simulink model "hdv_hydroelectropowertrain_model"  (R2023b)
settings: Solver=ode1be  StartTime=0.0  StopTime=simulation_length  FixedStep=tsample  MaxStep=tsample
values from neighbouring files (symbols this model uses):
  alpha = 35    [init_model.m]
  Apump = [0 1; 0 0]    [init_model.m]
  available_torque = torque_base+torque_friction_base    [init_model.m]
  Bpump = [0 1]'    [init_model.m]
  btheta_shaft = 2e2    (= 200)    [init_model.m]
  C1 = 10    [init_model.m]
  consumption = [consumption_1, consumption_2, consumption_3, consumption_4,          consumption_5, consumption_6, consumption_7, consumption_8,          consumption_9, consumption_10, consumption_11, consumption_12,          consumption_13, consumption_14, consumption_15, consumption_16          ]    [ic_engine_data.m]
  Cpump = [k 0]    [init_model.m]
  dp_lim = 400    [init_model.m]
  E0 = 3.685    [init_model.m]
  E1 = 0.2156    [init_model.m]
  E2 = 0    [init_model.m]
  E3 = 0    [init_model.m]
  E_1 = -1.031    [init_model.m]
  Elog = -0.05    [init_model.m]
  eta_v_m = 0.98    [init_model.m]
  eta_v_p = 0.97    [init_model.m]
  ki_dp_comp = 1/dp_lim    (= 0.0025)    [init_model.m]
  ki_te_comp = 2/te_lim    [init_model.m]
  kp_ctrl_m = 1    [init_model.m]
  kp_dp_comp = 0.5/dp_lim    (= 0.00125)    [init_model.m]
  kp_te_comp = 1/te_lim    [init_model.m]
  Kpump = acker(Apump,Bpump,poles)    [init_model.m]
  load_blade_enable = 0    [init_model.m]
  Lpump = acker(Apump',Cpump',pole_so)'    [init_model.m]
  M = 125    [init_model.m]
  Ncell = 185    [init_model.m]
  Npump = -1/(Cpump*inv(Apump-Bpump*Kpump)*Bpump)    [init_model.m]
  omega_e_rpm_ref = 1700    [init_model.m]
  omega_l_max_rpm = omega_l_max/(2*pi)*60    (= 50.3075969543)    [init_model.m]
  q1Kalman = tsample^2*1e-2    (= 1e-08)    [init_model.m]
  q2Kalman = tsample^1*1e-1    (= 0.0001)    [init_model.m]
  q3Kalman = 0    [init_model.m]
  Qhr = 400    [init_model.m]
  R0 = 0.015    [init_model.m]
  R1 = 0.015    [init_model.m]
  R_tg = 1.16/2    (= 0.58)    [init_model.m]
  rKalman = 1    [init_model.m]
  rpm_base = [620 700 800 900 1000 1100 1200 1300 1400 1500 1600 1700 1800      1900 2000 2100]    [ic_engine_data.m]
  rpm_consumption = rpm_base    [ic_engine_data.m]
  simulation_length = 245    [init_model.m]
  tau_load = 75e3    (= 75000)    [init_model.m]
  tau_load_max = 1600*41.4    (= 66240)    [init_model.m]
  Tc = tsample    (= 0.001)    [init_model.m]
  torque_base = [max(torque_16_data) max(torque_15_data) max(torque_14_data)      max(torque_13_data) max(torque_12_data) max(torque_11_data)      max(torque_10_data) max(torque_9_data) max(torque_8_data)      max(torque_7_data) max(torque_6_data) max(torque_5_data)      max(torque_4_data) max(torque_3_data) max(torque_2_data)      max(torque_1_data)]    [ic_engine_data.m]
  torque_consumption = torque_reference    [ic_engine_data.m]
  torque_friction_base = -(rpm_base./60*2*pi)*0.25-(rpm_base./60*2*pi).^2*5.2e-4    [ic_engine_data.m]
  tsample = 1e-3    (= 0.001)    [init_model.m]
  v_track1_ref = 8    [init_model.m]
  v_track2_ref = 8    [init_model.m]
  valve_mmorifice_max = 2.75    [init_model.m]
  xv_m_max = 1.2    [init_model.m]
undefined symbols (not defined in the file or in its folder): magnitude
libraries: fl_lib x381, nesl_utility x162, linear_swashplate_ctrl_lib x8, flexshaft_lib x5, bichamber_piston_lib x5, variable_displacement_motor_lib x4, variable_displacement_pump_lib x4, fixed_displacement_pump_lib x4, relief_valve_lib x4, inverse_shuttle_valve_lib x4, hydrostatic_threeway_valve_bichamber_piston_lib x4, hydrostatic_fourway_valve_bichamber_piston_lib x4
(part 2 of 9)

== system hdv_hydroelectropowertrain_model/Vehicle Control System/direction_lineLT ==
  In1 : Inport
  Abs1 : Abs  SaturateOnIntegerOverflow=off
  Product : Product
  Out1 : Outport
  wires:
  [direction_LT] -> Product/2
  In1/1 -> Abs1/1
  Product/1 -> Out1/1
  Abs1/1 -> Product/1

== system hdv_hydroelectropowertrain_model/Vehicle Control System/direction_lineRT ==
  In1 : Inport
  Abs : Abs  SaturateOnIntegerOverflow=off
  Product : Product
  Out1 : Outport
  wires:
  Product/1 -> Out1/1
  In1/1 -> Abs/1
  [direction_RT] -> Product/2
  Abs/1 -> Product/1

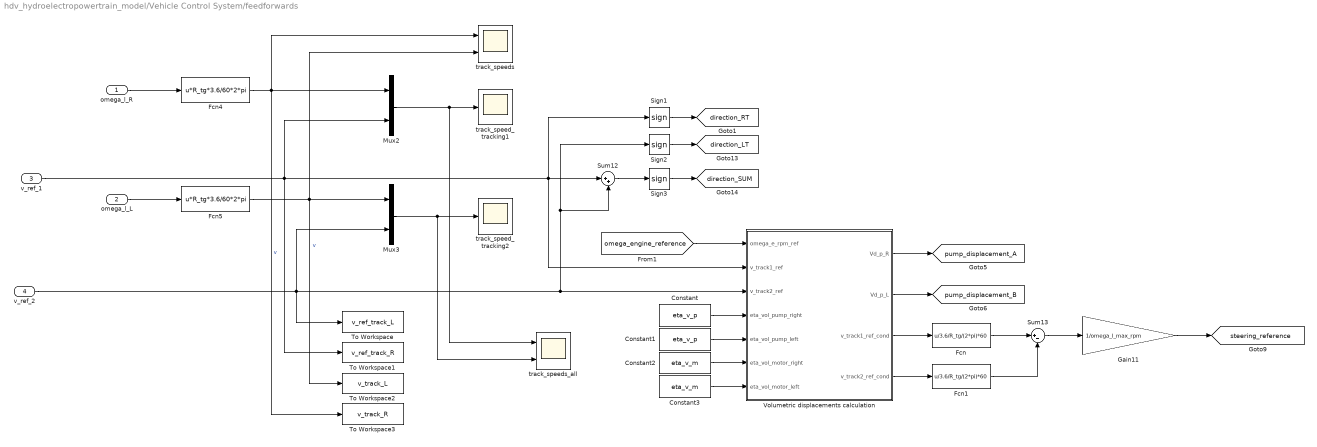
== system hdv_hydroelectropowertrain_model/Vehicle Control System/feedforwards ==
  omega_l_R : Inport
  omega_l_L : Inport  Port=2
  v_ref_1 : Inport  Port=3
  v_ref_2 : Inport  Port=4
  Constant : Constant  Value=eta_v_p
  Constant1 : Constant  Value=eta_v_p
  Constant2 : Constant  Value=eta_v_m
  Constant3 : Constant  Value=eta_v_m
  Fcn : Fcn  Expr=u/3.6/R_tg/(2*pi)*60
  Fcn1 : Fcn  Expr=u/3.6/R_tg/(2*pi)*60
  Fcn4 : Fcn  Expr=u*R_tg*3.6/60*2*pi
  Fcn5 : Fcn  Expr=u*R_tg*3.6/60*2*pi
  Gain11 : Gain  Gain=1/omega_l_max_rpm
  Mux2 : Mux  Inputs=2
  Mux3 : Mux  Inputs=2
  Sign1 : Signum
  Sign2 : Signum
  Sign3 : Signum
  Sum12 : Sum  Inputs=|++
  Sum13 : Sum  Inputs=|+-
  To Workspace : ToWorkspace  VariableName=v_ref_track_L  SampleTime=Tc
      settings: MaxDataPoints=Nc
  To Workspace1 : ToWorkspace  VariableName=v_ref_track_R  SampleTime=Tc
      settings: MaxDataPoints=Nc
  To Workspace2 : ToWorkspace  VariableName=v_track_L  SampleTime=Tc
      settings: MaxDataPoints=Nc
  To Workspace3 : ToWorkspace  VariableName=v_track_R  SampleTime=Tc
      settings: MaxDataPoints=Nc
  Volumetric displacements calculation : MATLAB Function  TreatAsAtomicUnit=on
  track_speed_tracking1 : Scope
  track_speed_tracking2 : Scope
  track_speeds : Scope  NumInputPorts=2
  track_speeds_all : Scope  NumInputPorts=2
  tag scope: direction_LT=global, direction_RT=global, direction_SUM=global, pump_displacement_A=global, pump_displacement_B=global, steering_reference=global
  wires:
  Constant3/1 -> Volumetric displacements calculation/7(eta_vol_motor_left)
  [omega_engine_reference] -> Volumetric displacements calculation/1(omega_e_rpm_ref)
  v_ref_2/1 -> To Workspace/1, Sign2/1, Sum12/2, Volumetric displacements calculation/3(v_track2_ref), Mux3/2
  v_ref_1/1 -> Mux2/2, To Workspace1/1, Volumetric displacements calculation/2(v_track1_ref), Sum12/1, Sign1/1
  Fcn/1 -> Sum13/1
  Constant/1 -> Volumetric displacements calculation/4(eta_vol_pump_right)
  Volumetric displacements calculation/4(v_track2_ref_cond) -> Fcn1/1
  Fcn5/1 -> To Workspace2/1, Mux3/1, track_speeds/2  "v"
  Constant1/1 -> Volumetric displacements calculation/5(eta_vol_pump_left)
  Sum13/1 -> Gain11/1
  Volumetric displacements calculation/3(v_track1_ref_cond) -> Fcn/1
  Sign1/1 -> [direction_RT]
  Fcn4/1 -> Mux2/1, track_speeds/1, To Workspace3/1  "v"
  Volumetric displacements calculation/1(Vd_p_R) -> [pump_displacement_A]
  Volumetric displacements calculation/2(Vd_p_L) -> [pump_displacement_B]
  omega_l_R/1 -> Fcn4/1
  Gain11/1 -> [steering_reference]
  Sign2/1 -> [direction_LT]
  Sum12/1 -> Sign3/1
  Sign3/1 -> [direction_SUM]
  Constant2/1 -> Volumetric displacements calculation/6(eta_vol_motor_right)
  Mux3/1 -> track_speeds_all/2, track_speed_tracking2/1
  Fcn1/1 -> Sum13/2
  Mux2/1 -> track_speeds_all/1, track_speed_tracking1/1
  omega_l_L/1 -> Fcn5/1

== system hdv_hydroelectropowertrain_model/Vehicle Control System/lineA_compensations ==
  Abs : Abs  SaturateOnIntegerOverflow=off
  Gain7 : Gain  Gain=-1
  Saturation Dynamic : simulink/Discontinuities/Saturation Dynamic  OutMin=[]  OutMax=[]  OutDataTypeStr=Inherit: Same as second input  OutDataType=fixdt(1, 16)  OutScaling=2^-10  DoSatur=off
  Sum13 : Sum  Inputs=++|
  compRT : Scope  NumInputPorts=2
  direction_RT : Subsystem
  displacement_compensation : Outport
  wires:
  Saturation Dynamic/1 -> displacement_compensation/1
  Sum13/1 -> Saturation Dynamic/2
  Gain7/1 -> compRT/2, Saturation Dynamic/3
  [compensation_pressureA] -> Sum13/1
  [compensation_engine] -> direction_RT/1(In1)
  direction_RT/1(ETComp) -> Sum13/2  "engine torque compensation"
  [pump_displacement_A] -> Abs/1
  Abs/1 -> Saturation Dynamic/1, compRT/1, Gain7/1

== system hdv_hydroelectropowertrain_model/Vehicle Control System/lineB_compensations  ==
  Abs : Abs  SaturateOnIntegerOverflow=off
  Gain7 : Gain  Gain=-1
  Saturation Dynamic : simulink/Discontinuities/Saturation Dynamic  OutMin=[]  OutMax=[]  OutDataTypeStr=Inherit: Same as second input  OutDataType=fixdt(1, 16)  OutScaling=2^-10  DoSatur=off
  Sum12 : Sum  Inputs=|++
  compLT : Scope  NumInputPorts=2
  direction_LT : Subsystem
  displacement_compensation : Outport
  wires:
  [compensation_pressureB] -> Sum12/2
  Gain7/1 -> compLT/2, Saturation Dynamic/3
  [compensation_engine] -> direction_LT/1(In1)
  direction_LT/1(ETComp) -> Sum12/1  "engine torque compensation"
  [pump_displacement_B] -> Abs/1
  Sum12/1 -> Saturation Dynamic/2
  Saturation Dynamic/1 -> displacement_compensation/1
  Abs/1 -> Saturation Dynamic/1, compLT/1, Gain7/1

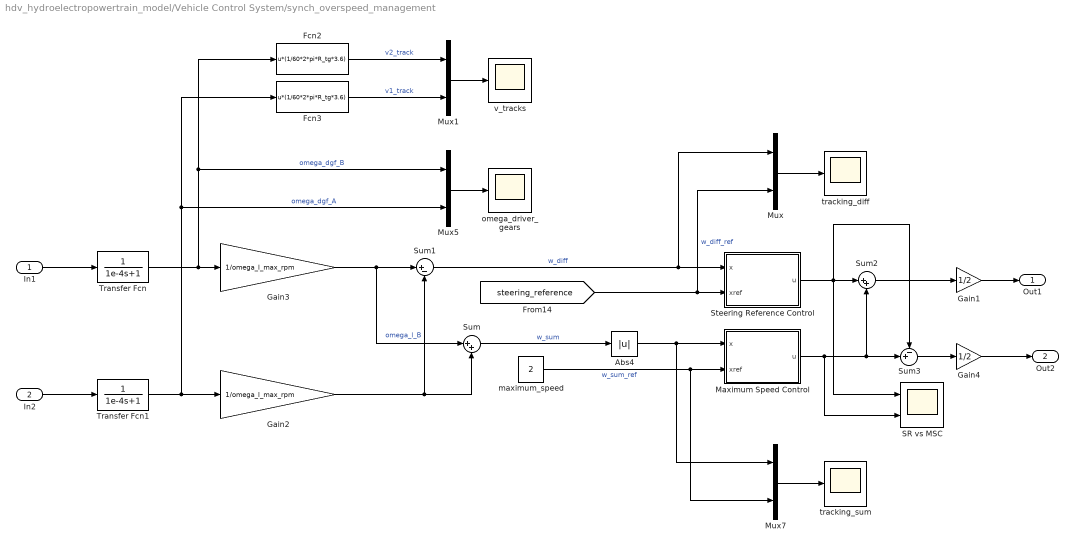
== system hdv_hydroelectropowertrain_model/Vehicle Control System/synch_overspeed_management ==
  In1 : Inport
  In2 : Inport  Port=2
  Abs4 : Abs  SaturateOnIntegerOverflow=off
  Fcn2 : Fcn  Expr=u*(1/60*2*pi*R_tg*3.6)
  Fcn3 : Fcn  Expr=u*(1/60*2*pi*R_tg*3.6)
  Gain1 : Gain  Gain=1/2
  Gain2 : Gain  Gain=1/omega_l_max_rpm
  Gain3 : Gain  Gain=1/omega_l_max_rpm
  Gain4 : Gain  Gain=1/2
  Maximum Speed Control : Subsystem  mask{kp=0.25/2, ki=4/2, ts=tsample, sat_pos=0, sat_neg=-3.28}
  Mux{,1,5,7} (4 alike) : Mux  Inputs=2
  SR vs MSC : Scope  NumInputPorts=2
  Steering Reference Control : Subsystem  mask{kp=0.125 %0.5, ki=2 %8, ts=tsample, sat_pos=3.28, sat_neg=-3.28}
  Sum : Sum  Inputs=|++
  Sum1 : Sum  Inputs=|+-
  Sum2 : Sum  Inputs=|++
  Sum3 : Sum  Inputs=-+|
  Transfer Fcn : TransferFcn  Denominator=[1e-4 1]
  Transfer Fcn1 : TransferFcn  Denominator=[1e-4 1]
  maximum_speed : Constant  Value=2
  omega_driver_gears : Scope
  tracking_diff : Scope
  tracking_sum : Scope
  v_tracks : Scope
  Out1 : Outport
  Out2 : Outport  Port=2
  wires:
  Mux7/1 -> tracking_sum/1
  Sum/1 -> Abs4/1  "w_sum"
  Gain3/1 -> Sum/1, Sum1/1
  Mux1/1 -> v_tracks/1
  maximum_speed/1 -> Maximum Speed Control/2(xref), Mux7/2  "w_sum_ref"
  Sum3/1 -> Gain4/1
  Sum1/1 -> Mux/1, Steering Reference Control/1(x)  "w_diff"
  Transfer Fcn/1 -> Fcn2/1, Mux5/1, Gain3/1  "omega_dgf_B"
  Maximum Speed Control/1(u) -> SR vs MSC/2, Sum2/2, Sum3/2
  Gain2/1 -> Sum1/2, Sum/2  "omega_l_B"
  In1/1 -> Transfer Fcn/1
  Mux/1 -> tracking_diff/1
  Gain1/1 -> Out1/1
  Sum2/1 -> Gain1/1
  Mux5/1 -> omega_driver_gears/1
  Abs4/1 -> Mux7/1, Maximum Speed Control/1(x)
  Fcn3/1 -> Mux1/2  "v1_track"
  [steering_reference] -> Mux/2, Steering Reference Control/2(xref)  "w_diff_ref"
  Steering Reference Control/1(u) -> Sum3/1, SR vs MSC/1, Sum2/1
  Transfer Fcn1/1 -> Fcn3/1, Mux5/2, Gain2/1  "omega_dgf_A"
  Fcn2/1 -> Mux1/1  "v2_track"
  Gain4/1 -> Out2/1
  In2/1 -> Transfer Fcn1/1

== system hdv_hydroelectropowertrain_model/Vehicle Control System/tracks references ==
  Manual Switch : ManualSwitch
  Manual Switch1 : ManualSwitch  CurrentSetting=0
  Repeating Sequence Stair1 : simulink/Sources/Repeating Sequence Stair  OutValues=[v_track2_ref -v_track2_ref v_track2_ref -v_track2_ref v_track2_ref -v_track2_ref].'  tsamp=floor(simulation_length/6)  OutMin=[]  OutMax=[]  OutDataTypeStr=double  OutputDataTypeScalingMode=double  OutDataType=fixdt(0,8)  ConRadixGroup=Best Precision: Vector-wise  OutScaling=2^-12
  Repeating Sequence Stair2 : simulink/Sources/Repeating Sequence Stair  OutValues=[v_track1_ref -v_track1_ref v_track1_ref -v_track1_ref v_track1_ref -v_track1_ref].'  tsamp=floor(simulation_length/6)  OutMin=[]  OutMax=[]  OutDataTypeStr=double  OutputDataTypeScalingMode=double  OutDataType=fixdt(0,8)  ConRadixGroup=Best Precision: Vector-wise  OutScaling=2^-12
  Sum : Sum  Inputs=|++
  Sum1 : Sum  Inputs=++|
  v_track1_ref : Step  Time=10  After=v_track1_ref  SampleTime=0
  v_track1_ref1 : Step  Time=simulation_length/2  After=-2*v_track1_ref  SampleTime=0
  v_track2_ref : Step  Time=10  After=v_track2_ref  SampleTime=0
  v_track2_ref1 : Step  Time=simulation_length/2  After=-2*v_track2_ref  SampleTime=0
  speed_track_1_ref : Outport
  speed_track_2_ref : Outport  Port=2
  wires:
  v_track1_ref1/1 -> Sum1/1
  v_track2_ref1/1 -> Sum/2
  v_track1_ref/1 -> Sum1/2
  v_track2_ref/1 -> Sum/1
  Manual Switch/1 -> speed_track_1_ref/1
  Manual Switch1/1 -> speed_track_2_ref/1
  Sum1/1 -> Manual Switch/2
  Sum/1 -> Manual Switch1/1
  Repeating Sequence Stair2/1 -> Manual Switch/1
  Repeating Sequence Stair1/1 -> Manual Switch1/2

== system hdv_hydroelectropowertrain_model/external_load/loadA ==
  Rate Limiter : RateLimiter  RisingSlewLimit=tau_load_max/5  FallingSlewLimit=-tau_load_max/5  SampleTimeMode=inherited
  Saturation : Saturate  UpperLimit=abs(tau_load)  LowerLimit=-abs(tau_load)
  Step : Step  Time=5  After=tau_load  SampleTime=0
  Out1 : Outport
  wires:
  Saturation/1 -> Out1/1
  Rate Limiter/1 -> Saturation/1
  Step/1 -> Rate Limiter/1

== system hdv_hydroelectropowertrain_model/external_load/loadB ==
  Rate Limiter : RateLimiter  RisingSlewLimit=tau_load_max/5  FallingSlewLimit=-tau_load_max/5  SampleTimeMode=inherited
  Saturation : Saturate  UpperLimit=abs(tau_load)  LowerLimit=-abs(tau_load)
  Step : Step  Time=5  After=tau_load  SampleTime=0
  Out1 : Outport
  wires:
  Step/1 -> Rate Limiter/1
  Rate Limiter/1 -> Saturation/1
  Saturation/1 -> Out1/1

== system hdv_hydroelectropowertrain_model/PR776_powertrain/Hydrostatic_powertrain/driveine_LD1 ==
  Connection Label1 : ConnectionLabel  Label=pS1
  Connection Label2 : ConnectionLabel  Label=pS1
  Connection Label3 : ConnectionLabel  Label=pT1
  Connection Label4 : ConnectionLabel  Label=pS2
  Connection Label5 : ConnectionLabel  Label=pT2
  Connection Label6 : ConnectionLabel  Label=pT1
  Connection Label7 : ConnectionLabel  Label=pS2
  Connection Label8 : ConnectionLabel  Label=pT2
  Variable displacement motor LD : variable_displacement_motor_lib/Variable displacement motor  max_Dv=Vm_nom cm^3/rev  min_Dv=20 cm^3/rev  inertia_motor=0.0402 kg*m^2  oil_vol=4.1 l  bp=b1 N*m/(rad/s)  lk=1e-6 m  t_specify=off  t_priority=None  t=0 N*m  t_nominal_specify=off  t_nominal_unit=N*m  t_nominal_value=1  q_specify=off  q_priority=None  q=0 m^3/s  q_nominal_specify=off  q_nominal_unit=m^3/s  q_nominal_value=1  qt_specify=off  qt_priority=None  qt=0 m^3/s  qt_nominal_specify=off  qt_nominal_unit=m^3/s  qt_nominal_value=1  qleak_specify=off  qleak_priority=None  qleak=0 m^3/s  qleak_nominal_specify=off  qleak_nominal_unit=m^3/s  qleak_nominal_value=1  Dv_specify=off  Dv_priority=None  Dv=0 cm^3/rev  Dv_nominal_specify=off  Dv_nominal_unit=cm^3/rev  Dv_nominal_value=1  dp_specify=off  dp_priority=None  dp=0 Pa  dp_nominal_specify=off  dp_nominal_unit=Pa  dp_nominal_value=1  wm_specify=off  wm_priority=None  wm=0 rad/s  wm_nominal_specify=off  wm_nominal_unit=rad/s  wm_nominal_value=1
      settings: InternalSimscapePortConfiguration="{\"Bottom\":[],\"Left\":[{\"id\":\"Vd\",\"label\":\"Vd\",\"type\":\"input\"},{\"id\":\"A\",\"label\":\"A\",\"type\":\"foundation.hydraulic.hydraulic\"},{\"id\":\"B\",\"label\":\"B\",\"type\":\"foundation.hydraulic.hydraulic\"}],\"Right\":[{\"id\":\"C\",\"label\":\"C\",\"type\":\"foundation.mechanical.rotational.rotational\"},{\"id\":\"q_out\",\"label\":\"q\",\"type\":\"output\"},{\"id\":\"delta_p_out\",\"label\":\"dp\",\"type\":\"output\"}],\"Top\":[]}"
  Variable displacement pump LD : variable_displacement_pump_lib/Variable displacement pump  max_Dv=Vp_nom cm^3/rev  inertia_pump=0.027 kg*m^2  oil_vol=3.0 l  bp=b1 N*m/(rad/s)  lk=1e-6 m  t_specify=off  t_priority=None  t=0 N*m  t_nominal_specify=off  t_nominal_unit=N*m  t_nominal_value=1  q_specify=off  q_priority=None  q=0 m^3/s  q_nominal_specify=off  q_nominal_unit=m^3/s  q_nominal_value=1  qt_specify=off  qt_priority=None  qt=0 m^3/s  qt_nominal_specify=off  qt_nominal_unit=m^3/s  qt_nominal_value=1  qleak_specify=off  qleak_priority=None  qleak=0 m^3/s  qleak_nominal_specify=off  qleak_nominal_unit=m^3/s  qleak_nominal_value=1  Dv_specify=off  Dv_priority=None  Dv=0 cm^3/rev  Dv_nominal_specify=off  Dv_nominal_unit=cm^3/rev  Dv_nominal_value=1  dp_specify=off  dp_priority=None  dp=0 Pa  dp_nominal_specify=off  dp_nominal_unit=Pa  dp_nominal_value=1  we_specify=off  we_priority=None  we=0 rad/s  we_nominal_specify=off  we_nominal_unit=rad/s  we_nominal_value=1
      settings: InternalSimscapePortConfiguration="{\"Bottom\":[],\"Left\":[{\"id\":\"Vd\",\"label\":\"Vd\",\"type\":\"input\"},{\"id\":\"C\",\"label\":\"C\",\"type\":\"foundation.mechanical.rotational.rotational\"}],\"Right\":[{\"id\":\"A\",\"label\":\"A\",\"type\":\"foundation.hydraulic.hydraulic\"},{\"id\":\"B\",\"label\":\"B\",\"type\":\"foundation.hydraulic.hydraulic\"}],\"Top\":[]}"
  flexible shaft1 : flexshaft_lib/flexible shaft  b1=b1 N*m/(rad/s)  J1=J1 kg*m^2  b2=b2 N*m/(rad/s)  J2=J2 kg*m^2  b_theta=b_theta N*m/(rad/s)  k_theta=k_theta N*m/rad  w_1_specify=off  w_1_priority=None  w_1=0 rad/s  w_1_nominal_specify=off  w_1_nominal_unit=rad/s  w_1_nominal_value=1  w_2_specify=off  w_2_priority=None  w_2=0 rad/s  w_2_nominal_specify=off  w_2_nominal_unit=rad/s  w_2_nominal_value=1  t_1_specify=off  t_1_priority=None  t_1=0 N*m  t_1_nominal_specify=off  t_1_nominal_unit=N*m  t_1_nominal_value=1  t_2_specify=off  t_2_priority=None  t_2=0 N*m  t_2_nominal_specify=off  t_2_nominal_unit=N*m  t_2_nominal_value=1  t_theta_specify=off  t_theta_priority=None  t_theta=0 N*m  t_theta_nominal_specify=off  t_theta_nominal_unit=N*m  t_theta_nominal_value=1
      settings: InternalSimscapePortConfiguration="{\"Bottom\":[],\"Left\":[{\"id\":\"S1\",\"label\":\"S1\",\"type\":\"foundation.mechanical.rotational.rotational\"}],\"Right\":[{\"id\":\"S2\",\"label\":\"S2\",\"type\":\"foundation.mechanical.rotational.rotational\"},{\"id\":\"tau2\",\"label\":\"tau2\",\"type\":\"output\"},{\"id\":\"w2\",\"label\":\"w2\",\"type\":\"output\"}],\"Top\":[]}"
  pressure_charge_system_LD : Subsystem
      settings: PortSchema="{\"entries\":[{\"content\":{\"sides\":[{\"content\":{\"connectorIds\":[]},\"type\":\"ConnectorPlacement.EquallySpacedRectSide\",\"uuid\":\"e48dc60c-7abd-410a-894b-273047c8aadd\"},{\"content\":{\"connectorIds\":[],\"side\":\"RIGHT\"},\"type\":\"ConnectorPlacement.EquallySpacedRectSide\",\"uuid\":\"1866d745-b28e-4187-be81-03bff766c239\"},{\"content\":{\"connectorIds\":[\"LConn1\"],\"side\":\"TOP\"},\"type\":\"ConnectorPlacement.EquallySpacedRectSide\",\"uuid\":\"a7856f22-1a7f-4c46-a37a-59c4b01a6b79\"},{\"content\":{\"connectorIds\":[\"RConn1\",\"RConn2\"],\"side\":\"BOTTOM\"},\"type\":\"ConnectorPlacement.EquallySpacedRectSide\",\"uuid\":\"6254cc6e-0892-4919-86d5-0180151530d1\"}]},\"type\":\"ConnectorPlacement.EquallySpacedConnector\",\"uuid\":\"a983534e-afc0-4bb2-9b1c-06b03353b26b\"}],\"packageUris\":[\"http://schema.mathworks.com/mf0/Connector/19700101\"],\"version\":\"1.0\"}"
  vd_ctrl_motor_LD : Subsystem
  vd_ctrl_pump_LD : Subsystem
  s : PMIOPort  Side=Left
  pS1 : PMIOPort  Port=2  Side=Left
  pS2 : PMIOPort  Port=3  Side=Left
  pT1 : PMIOPort  Port=4  Side=Left
  pT2 : PMIOPort  Port=5  Side=Left
  q : PMIOPort  Port=6  Side=Right
  dp : PMIOPort  Port=7  Side=Right
  c : PMIOPort  Port=8  Side=Right
  RDA : PMIOPort  Port=9  Side=Right
  RDB : PMIOPort  Port=10  Side=Right
  wires:
  [DpB] -> vd_ctrl_pump_LD/1(vd_ref)
  [DmB] -> vd_ctrl_motor_LD/1(vd_ref)
  connections:
  flexible shaft1/LConn1 -- s/RConn1
  Variable displacement pump LD/RConn1 -- RDA/RConn1 -- Variable displacement motor LD/LConn2 -- pressure_charge_system_LD/LConn1
  vd_ctrl_pump_LD/RConn1 -- Variable displacement pump LD/LConn1
  vd_ctrl_pump_LD/LConn1 -- Connection Label2/LConn1
  flexible shaft1/RConn1 -- pressure_charge_system_LD/RConn2 -- Variable displacement pump LD/LConn2
  vd_ctrl_motor_LD/RConn1 -- Variable displacement motor LD/LConn1
  vd_ctrl_pump_LD/LConn2 -- Connection Label3/LConn1
  Connection Label4/LConn1 -- vd_ctrl_motor_LD/LConn1
  Connection Label5/LConn1 -- vd_ctrl_motor_LD/LConn2
  Variable displacement motor LD/LConn3 -- pressure_charge_system_LD/RConn1 -- Variable displacement pump LD/RConn2 -- RDB/RConn1
  Variable displacement motor LD/RConn2 -- q/RConn1
  Variable displacement motor LD/RConn3 -- dp/RConn1
  c/RConn1 -- Variable displacement motor LD/RConn1
  pS2/RConn1 -- Connection Label7/LConn1
  pS1/RConn1 -- Connection Label1/LConn1
  pT1/RConn1 -- Connection Label6/LConn1
  pT2/RConn1 -- Connection Label8/LConn1

== system hdv_hydroelectropowertrain_model/PR776_powertrain/Hydrostatic_powertrain/driveine_LD2 ==
  Connection Label1 : ConnectionLabel  Label=pS1
  Connection Label2 : ConnectionLabel  Label=pS1
  Connection Label3 : ConnectionLabel  Label=pT1
  Connection Label4 : ConnectionLabel  Label=pS2
  Connection Label5 : ConnectionLabel  Label=pT2
  Connection Label6 : ConnectionLabel  Label=pT1
  Connection Label7 : ConnectionLabel  Label=pS2
  Connection Label8 : ConnectionLabel  Label=pT2
  Variable displacement motor LD : variable_displacement_motor_lib/Variable displacement motor  max_Dv=Vm_nom cm^3/rev  min_Dv=20 cm^3/rev  inertia_motor=0.0402 kg*m^2  oil_vol=4.1 l  bp=b1 N*m/(rad/s)  lk=1e-6 m  t_specify=off  t_priority=None  t=0 N*m  t_nominal_specify=off  t_nominal_unit=N*m  t_nominal_value=1  q_specify=off  q_priority=None  q=0 m^3/s  q_nominal_specify=off  q_nominal_unit=m^3/s  q_nominal_value=1  qt_specify=off  qt_priority=None  qt=0 m^3/s  qt_nominal_specify=off  qt_nominal_unit=m^3/s  qt_nominal_value=1  qleak_specify=off  qleak_priority=None  qleak=0 m^3/s  qleak_nominal_specify=off  qleak_nominal_unit=m^3/s  qleak_nominal_value=1  Dv_specify=off  Dv_priority=None  Dv=0 cm^3/rev  Dv_nominal_specify=off  Dv_nominal_unit=cm^3/rev  Dv_nominal_value=1  dp_specify=off  dp_priority=None  dp=0 Pa  dp_nominal_specify=off  dp_nominal_unit=Pa  dp_nominal_value=1  wm_specify=off  wm_priority=None  wm=0 rad/s  wm_nominal_specify=off  wm_nominal_unit=rad/s  wm_nominal_value=1
      settings: InternalSimscapePortConfiguration="{\"Bottom\":[],\"Left\":[{\"id\":\"Vd\",\"label\":\"Vd\",\"type\":\"input\"},{\"id\":\"A\",\"label\":\"A\",\"type\":\"foundation.hydraulic.hydraulic\"},{\"id\":\"B\",\"label\":\"B\",\"type\":\"foundation.hydraulic.hydraulic\"}],\"Right\":[{\"id\":\"C\",\"label\":\"C\",\"type\":\"foundation.mechanical.rotational.rotational\"},{\"id\":\"q_out\",\"label\":\"q\",\"type\":\"output\"},{\"id\":\"delta_p_out\",\"label\":\"dp\",\"type\":\"output\"}],\"Top\":[]}"
  Variable displacement pump LD : variable_displacement_pump_lib/Variable displacement pump  max_Dv=Vp_nom cm^3/rev  inertia_pump=0.027 kg*m^2  oil_vol=3.0 l  bp=b1 N*m/(rad/s)  lk=1e-6 m  t_specify=off  t_priority=None  t=0 N*m  t_nominal_specify=off  t_nominal_unit=N*m  t_nominal_value=1  q_specify=off  q_priority=None  q=0 m^3/s  q_nominal_specify=off  q_nominal_unit=m^3/s  q_nominal_value=1  qt_specify=off  qt_priority=None  qt=0 m^3/s  qt_nominal_specify=off  qt_nominal_unit=m^3/s  qt_nominal_value=1  qleak_specify=off  qleak_priority=None  qleak=0 m^3/s  qleak_nominal_specify=off  qleak_nominal_unit=m^3/s  qleak_nominal_value=1  Dv_specify=off  Dv_priority=None  Dv=0 cm^3/rev  Dv_nominal_specify=off  Dv_nominal_unit=cm^3/rev  Dv_nominal_value=1  dp_specify=off  dp_priority=None  dp=0 Pa  dp_nominal_specify=off  dp_nominal_unit=Pa  dp_nominal_value=1  we_specify=off  we_priority=None  we=0 rad/s  we_nominal_specify=off  we_nominal_unit=rad/s  we_nominal_value=1
      settings: InternalSimscapePortConfiguration="{\"Bottom\":[],\"Left\":[{\"id\":\"Vd\",\"label\":\"Vd\",\"type\":\"input\"},{\"id\":\"C\",\"label\":\"C\",\"type\":\"foundation.mechanical.rotational.rotational\"}],\"Right\":[{\"id\":\"A\",\"label\":\"A\",\"type\":\"foundation.hydraulic.hydraulic\"},{\"id\":\"B\",\"label\":\"B\",\"type\":\"foundation.hydraulic.hydraulic\"}],\"Top\":[]}"
  flexible shaft1 : flexshaft_lib/flexible shaft  b1=b1 N*m/(rad/s)  J1=J1 kg*m^2  b2=b2 N*m/(rad/s)  J2=J2 kg*m^2  b_theta=b_theta N*m/(rad/s)  k_theta=k_theta N*m/rad  w_1_specify=off  w_1_priority=None  w_1=0 rad/s  w_1_nominal_specify=off  w_1_nominal_unit=rad/s  w_1_nominal_value=1  w_2_specify=off  w_2_priority=None  w_2=0 rad/s  w_2_nominal_specify=off  w_2_nominal_unit=rad/s  w_2_nominal_value=1  t_1_specify=off  t_1_priority=None  t_1=0 N*m  t_1_nominal_specify=off  t_1_nominal_unit=N*m  t_1_nominal_value=1  t_2_specify=off  t_2_priority=None  t_2=0 N*m  t_2_nominal_specify=off  t_2_nominal_unit=N*m  t_2_nominal_value=1  t_theta_specify=off  t_theta_priority=None  t_theta=0 N*m  t_theta_nominal_specify=off  t_theta_nominal_unit=N*m  t_theta_nominal_value=1
      settings: InternalSimscapePortConfiguration="{\"Bottom\":[],\"Left\":[{\"id\":\"S1\",\"label\":\"S1\",\"type\":\"foundation.mechanical.rotational.rotational\"}],\"Right\":[{\"id\":\"S2\",\"label\":\"S2\",\"type\":\"foundation.mechanical.rotational.rotational\"},{\"id\":\"tau2\",\"label\":\"tau2\",\"type\":\"output\"},{\"id\":\"w2\",\"label\":\"w2\",\"type\":\"output\"}],\"Top\":[]}"
  pressure_charge_system_LD : Subsystem
      settings: PortSchema="{\"entries\":[{\"content\":{\"sides\":[{\"content\":{\"connectorIds\":[]},\"type\":\"ConnectorPlacement.EquallySpacedRectSide\",\"uuid\":\"e48dc60c-7abd-410a-894b-273047c8aadd\"},{\"content\":{\"connectorIds\":[],\"side\":\"RIGHT\"},\"type\":\"ConnectorPlacement.EquallySpacedRectSide\",\"uuid\":\"1866d745-b28e-4187-be81-03bff766c239\"},{\"content\":{\"connectorIds\":[\"LConn1\"],\"side\":\"TOP\"},\"type\":\"ConnectorPlacement.EquallySpacedRectSide\",\"uuid\":\"a7856f22-1a7f-4c46-a37a-59c4b01a6b79\"},{\"content\":{\"connectorIds\":[\"RConn1\",\"RConn2\"],\"side\":\"BOTTOM\"},\"type\":\"ConnectorPlacement.EquallySpacedRectSide\",\"uuid\":\"6254cc6e-0892-4919-86d5-0180151530d1\"}]},\"type\":\"ConnectorPlacement.EquallySpacedConnector\",\"uuid\":\"a983534e-afc0-4bb2-9b1c-06b03353b26b\"}],\"packageUris\":[\"http://schema.mathworks.com/mf0/Connector/19700101\"],\"version\":\"1.0\"}"
  vd_ctrl_motor_LD : Subsystem
  vd_ctrl_pump_LD : Subsystem
  s : PMIOPort  Side=Left
  pS1 : PMIOPort  Port=2  Side=Left
  pS2 : PMIOPort  Port=3  Side=Left
  pT1 : PMIOPort  Port=4  Side=Left
  pT2 : PMIOPort  Port=5  Side=Left
  q : PMIOPort  Port=6  Side=Right
  dp : PMIOPort  Port=7  Side=Right
  c : PMIOPort  Port=8  Side=Right
  RDA : PMIOPort  Port=9  Side=Right
  RDB : PMIOPort  Port=10  Side=Right
  wires:
  [DmB] -> vd_ctrl_motor_LD/1(vd_ref)
  [DpB] -> vd_ctrl_pump_LD/1(vd_ref)
  connections:
  pT2/RConn1 -- Connection Label8/LConn1
  pT1/RConn1 -- Connection Label6/LConn1
  pS1/RConn1 -- Connection Label1/LConn1
  pS2/RConn1 -- Connection Label7/LConn1
  c/RConn1 -- Variable displacement motor LD/RConn1
  Variable displacement motor LD/RConn3 -- dp/RConn1
  Variable displacement motor LD/RConn2 -- q/RConn1
  pressure_charge_system_LD/RConn1 -- Variable displacement motor LD/LConn3 -- RDB/RConn1 -- Variable displacement pump LD/RConn2
  Connection Label5/LConn1 -- vd_ctrl_motor_LD/LConn2
  Connection Label4/LConn1 -- vd_ctrl_motor_LD/LConn1
  vd_ctrl_pump_LD/LConn2 -- Connection Label3/LConn1
  vd_ctrl_motor_LD/RConn1 -- Variable displacement motor LD/LConn1
  Variable displacement pump LD/LConn2 -- pressure_charge_system_LD/RConn2 -- flexible shaft1/RConn1
  vd_ctrl_pump_LD/LConn1 -- Connection Label2/LConn1
  vd_ctrl_pump_LD/RConn1 -- Variable displacement pump LD/LConn1
  pressure_charge_system_LD/LConn1 -- RDA/RConn1 -- Variable displacement pump LD/RConn1 -- Variable displacement motor LD/LConn2
  flexible shaft1/LConn1 -- s/RConn1

== system hdv_hydroelectropowertrain_model/PR776_powertrain/Hydrostatic_powertrain/driveine_RD1 ==
  Connection Label1 : ConnectionLabel  Label=pS1
  Connection Label2 : ConnectionLabel  Label=pT1
  Connection Label3 : ConnectionLabel  Label=pS2
  Connection Label4 : ConnectionLabel  Label=pT2
  Connection Label6 : ConnectionLabel  Label=pS1
  Connection Label7 : ConnectionLabel  Label=pT1
  Connection Label8 : ConnectionLabel  Label=pS2
  Connection Label9 : ConnectionLabel  Label=pT2
  Variable displacement motor RD : variable_displacement_motor_lib/Variable displacement motor  max_Dv=Vm_nom cm^3/rev  min_Dv=20 cm^3/rev  inertia_motor=0.0402 kg*m^2  oil_vol=4.1 l  bp=b1 N*m/(rad/s)  lk=1e-6 m  t_specify=off  t_priority=None  t=0 N*m  t_nominal_specify=off  t_nominal_unit=N*m  t_nominal_value=1  q_specify=off  q_priority=None  q=0 m^3/s  q_nominal_specify=off  q_nominal_unit=m^3/s  q_nominal_value=1  qt_specify=off  qt_priority=None  qt=0 m^3/s  qt_nominal_specify=off  qt_nominal_unit=m^3/s  qt_nominal_value=1  qleak_specify=off  qleak_priority=None  qleak=0 m^3/s  qleak_nominal_specify=off  qleak_nominal_unit=m^3/s  qleak_nominal_value=1  Dv_specify=off  Dv_priority=None  Dv=0 cm^3/rev  Dv_nominal_specify=off  Dv_nominal_unit=cm^3/rev  Dv_nominal_value=1  dp_specify=off  dp_priority=None  dp=0 Pa  dp_nominal_specify=off  dp_nominal_unit=Pa  dp_nominal_value=1  wm_specify=off  wm_priority=None  wm=0 rad/s  wm_nominal_specify=off  wm_nominal_unit=rad/s  wm_nominal_value=1
      settings: InternalSimscapePortConfiguration="{\"Bottom\":[],\"Left\":[{\"id\":\"Vd\",\"label\":\"Vd\",\"type\":\"input\"},{\"id\":\"A\",\"label\":\"A\",\"type\":\"foundation.hydraulic.hydraulic\"},{\"id\":\"B\",\"label\":\"B\",\"type\":\"foundation.hydraulic.hydraulic\"}],\"Right\":[{\"id\":\"C\",\"label\":\"C\",\"type\":\"foundation.mechanical.rotational.rotational\"},{\"id\":\"q_out\",\"label\":\"q\",\"type\":\"output\"},{\"id\":\"delta_p_out\",\"label\":\"dp\",\"type\":\"output\"}],\"Top\":[]}"
  Variable displacement pump RD : variable_displacement_pump_lib/Variable displacement pump  max_Dv=Vp_nom cm^3/rev  inertia_pump=0.027 kg*m^2  oil_vol=3.0 l  bp=b1 N*m/(rad/s)  lk=1e-6 m  t_specify=off  t_priority=None  t=0 N*m  t_nominal_specify=off  t_nominal_unit=N*m  t_nominal_value=1  q_specify=off  q_priority=None  q=0 m^3/s  q_nominal_specify=off  q_nominal_unit=m^3/s  q_nominal_value=1  qt_specify=off  qt_priority=None  qt=0 m^3/s  qt_nominal_specify=off  qt_nominal_unit=m^3/s  qt_nominal_value=1  qleak_specify=off  qleak_priority=None  qleak=0 m^3/s  qleak_nominal_specify=off  qleak_nominal_unit=m^3/s  qleak_nominal_value=1  Dv_specify=off  Dv_priority=None  Dv=0 cm^3/rev  Dv_nominal_specify=off  Dv_nominal_unit=cm^3/rev  Dv_nominal_value=1  dp_specify=off  dp_priority=None  dp=0 Pa  dp_nominal_specify=off  dp_nominal_unit=Pa  dp_nominal_value=1  we_specify=off  we_priority=None  we=0 rad/s  we_nominal_specify=off  we_nominal_unit=rad/s  we_nominal_value=1
      settings: InternalSimscapePortConfiguration="{\"Bottom\":[],\"Left\":[{\"id\":\"Vd\",\"label\":\"Vd\",\"type\":\"input\"},{\"id\":\"C\",\"label\":\"C\",\"type\":\"foundation.mechanical.rotational.rotational\"}],\"Right\":[{\"id\":\"A\",\"label\":\"A\",\"type\":\"foundation.hydraulic.hydraulic\"},{\"id\":\"B\",\"label\":\"B\",\"type\":\"foundation.hydraulic.hydraulic\"}],\"Top\":[]}"
  flexible shaft2 : flexshaft_lib/flexible shaft  b1=b1 N*m/(rad/s)  J1=J1 kg*m^2  b2=b2 N*m/(rad/s)  J2=J2 kg*m^2  b_theta=b_theta N*m/(rad/s)  k_theta=k_theta N*m/rad  w_1_specify=off  w_1_priority=None  w_1=0 rad/s  w_1_nominal_specify=off  w_1_nominal_unit=rad/s  w_1_nominal_value=1  w_2_specify=off  w_2_priority=None  w_2=0 rad/s  w_2_nominal_specify=off  w_2_nominal_unit=rad/s  w_2_nominal_value=1  t_1_specify=off  t_1_priority=None  t_1=0 N*m  t_1_nominal_specify=off  t_1_nominal_unit=N*m  t_1_nominal_value=1  t_2_specify=off  t_2_priority=None  t_2=0 N*m  t_2_nominal_specify=off  t_2_nominal_unit=N*m  t_2_nominal_value=1  t_theta_specify=off  t_theta_priority=None  t_theta=0 N*m  t_theta_nominal_specify=off  t_theta_nominal_unit=N*m  t_theta_nominal_value=1
      settings: InternalSimscapePortConfiguration="{\"Bottom\":[],\"Left\":[{\"id\":\"S1\",\"label\":\"S1\",\"type\":\"foundation.mechanical.rotational.rotational\"}],\"Right\":[{\"id\":\"S2\",\"label\":\"S2\",\"type\":\"foundation.mechanical.rotational.rotational\"},{\"id\":\"tau2\",\"label\":\"tau2\",\"type\":\"output\"},{\"id\":\"w2\",\"label\":\"w2\",\"type\":\"output\"}],\"Top\":[]}"
  pressure_charge_system_RD : Subsystem
      settings: PortSchema="{\"entries\":[{\"content\":{\"sides\":[{\"content\":{\"connectorIds\":[]},\"type\":\"ConnectorPlacement.EquallySpacedRectSide\",\"uuid\":\"e48dc60c-7abd-410a-894b-273047c8aadd\"},{\"content\":{\"connectorIds\":[],\"side\":\"RIGHT\"},\"type\":\"ConnectorPlacement.EquallySpacedRectSide\",\"uuid\":\"1866d745-b28e-4187-be81-03bff766c239\"},{\"content\":{\"connectorIds\":[\"LConn1\"],\"side\":\"TOP\"},\"type\":\"ConnectorPlacement.EquallySpacedRectSide\",\"uuid\":\"a7856f22-1a7f-4c46-a37a-59c4b01a6b79\"},{\"content\":{\"connectorIds\":[\"RConn1\",\"RConn2\"],\"side\":\"BOTTOM\"},\"type\":\"ConnectorPlacement.EquallySpacedRectSide\",\"uuid\":\"6254cc6e-0892-4919-86d5-0180151530d1\"}]},\"type\":\"ConnectorPlacement.EquallySpacedConnector\",\"uuid\":\"a983534e-afc0-4bb2-9b1c-06b03353b26b\"}],\"packageUris\":[\"http://schema.mathworks.com/mf0/Connector/19700101\"],\"version\":\"1.0\"}"
  vd_ctrl_motor_RD : Subsystem
  vd_ctrl_pump_RD : Subsystem
  s : PMIOPort  Side=Left
  q : PMIOPort  Port=2  Side=Right
  dp : PMIOPort  Port=3  Side=Right
  c : PMIOPort  Port=4  Side=Right
  pS1 : PMIOPort  Port=5  Side=Left
  pS2 : PMIOPort  Port=6  Side=Left
  pT1 : PMIOPort  Port=7  Side=Left
  pT2 : PMIOPort  Port=8  Side=Left
  RDA : PMIOPort  Port=9  Side=Right
  RDB : PMIOPort  Port=10  Side=Right
  wires:
  [DmA] -> vd_ctrl_motor_RD/1(vd_ref)
  [DpA] -> vd_ctrl_pump_RD/1(vd_ref)
  connections:
  Variable displacement motor RD/LConn3 -- pressure_charge_system_RD/RConn1 -- RDB/RConn1 -- Variable displacement pump RD/RConn2
  Connection Label7/LConn1 -- vd_ctrl_pump_RD/LConn2
  flexible shaft2/RConn1 -- pressure_charge_system_RD/RConn2 -- Variable displacement pump RD/LConn2
  Connection Label6/LConn1 -- vd_ctrl_pump_RD/LConn1
  vd_ctrl_motor_RD/RConn1 -- Variable displacement motor RD/LConn1
  vd_ctrl_motor_RD/LConn2 -- Connection Label9/LConn1
  vd_ctrl_motor_RD/LConn1 -- Connection Label8/LConn1
  Variable displacement pump RD/RConn1 -- RDA/RConn1 -- Variable displacement motor RD/LConn2 -- pressure_charge_system_RD/LConn1
  vd_ctrl_pump_RD/RConn1 -- Variable displacement pump RD/LConn1
  s/RConn1 -- flexible shaft2/LConn1
  Variable displacement motor RD/RConn2 -- q/RConn1
  Variable displacement motor RD/RConn1 -- c/RConn1
  Variable displacement motor RD/RConn3 -- dp/RConn1
  pS1/RConn1 -- Connection Label1/LConn1
  pT1/RConn1 -- Connection Label2/LConn1
  pS2/RConn1 -- Connection Label3/LConn1
  pT2/RConn1 -- Connection Label4/LConn1

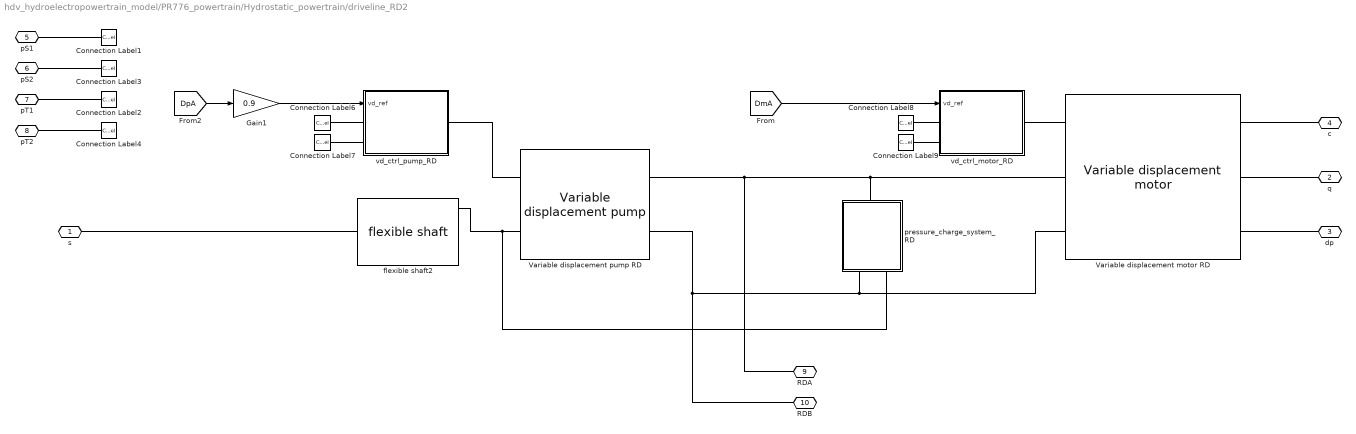
== system hdv_hydroelectropowertrain_model/PR776_powertrain/Hydrostatic_powertrain/driveline_RD2 ==
  Connection Label1 : ConnectionLabel  Label=pS1
  Connection Label2 : ConnectionLabel  Label=pT1
  Connection Label3 : ConnectionLabel  Label=pS2
  Connection Label4 : ConnectionLabel  Label=pT2
  Connection Label6 : ConnectionLabel  Label=pS1
  Connection Label7 : ConnectionLabel  Label=pT1
  Connection Label8 : ConnectionLabel  Label=pS2
  Connection Label9 : ConnectionLabel  Label=pT2
  Gain1 : Gain  Gain=0.9
  Variable displacement motor RD : variable_displacement_motor_lib/Variable displacement motor  max_Dv=Vm_nom cm^3/rev  min_Dv=20 cm^3/rev  inertia_motor=0.0402 kg*m^2  oil_vol=4.1 l  bp=b1 N*m/(rad/s)  lk=1e-6 m  t_specify=off  t_priority=None  t=0 N*m  t_nominal_specify=off  t_nominal_unit=N*m  t_nominal_value=1  q_specify=off  q_priority=None  q=0 m^3/s  q_nominal_specify=off  q_nominal_unit=m^3/s  q_nominal_value=1  qt_specify=off  qt_priority=None  qt=0 m^3/s  qt_nominal_specify=off  qt_nominal_unit=m^3/s  qt_nominal_value=1  qleak_specify=off  qleak_priority=None  qleak=0 m^3/s  qleak_nominal_specify=off  qleak_nominal_unit=m^3/s  qleak_nominal_value=1  Dv_specify=off  Dv_priority=None  Dv=0 cm^3/rev  Dv_nominal_specify=off  Dv_nominal_unit=cm^3/rev  Dv_nominal_value=1  dp_specify=off  dp_priority=None  dp=0 Pa  dp_nominal_specify=off  dp_nominal_unit=Pa  dp_nominal_value=1  wm_specify=off  wm_priority=None  wm=0 rad/s  wm_nominal_specify=off  wm_nominal_unit=rad/s  wm_nominal_value=1
      settings: InternalSimscapePortConfiguration="{\"Bottom\":[],\"Left\":[{\"id\":\"Vd\",\"label\":\"Vd\",\"type\":\"input\"},{\"id\":\"A\",\"label\":\"A\",\"type\":\"foundation.hydraulic.hydraulic\"},{\"id\":\"B\",\"label\":\"B\",\"type\":\"foundation.hydraulic.hydraulic\"}],\"Right\":[{\"id\":\"C\",\"label\":\"C\",\"type\":\"foundation.mechanical.rotational.rotational\"},{\"id\":\"q_out\",\"label\":\"q\",\"type\":\"output\"},{\"id\":\"delta_p_out\",\"label\":\"dp\",\"type\":\"output\"}],\"Top\":[]}"
  Variable displacement pump RD : variable_displacement_pump_lib/Variable displacement pump  max_Dv=Vp_nom cm^3/rev  inertia_pump=0.027 kg*m^2  oil_vol=3.0 l  bp=b1 N*m/(rad/s)  lk=1e-6 m  t_specify=off  t_priority=None  t=0 N*m  t_nominal_specify=off  t_nominal_unit=N*m  t_nominal_value=1  q_specify=off  q_priority=None  q=0 m^3/s  q_nominal_specify=off  q_nominal_unit=m^3/s  q_nominal_value=1  qt_specify=off  qt_priority=None  qt=0 m^3/s  qt_nominal_specify=off  qt_nominal_unit=m^3/s  qt_nominal_value=1  qleak_specify=off  qleak_priority=None  qleak=0 m^3/s  qleak_nominal_specify=off  qleak_nominal_unit=m^3/s  qleak_nominal_value=1  Dv_specify=off  Dv_priority=None  Dv=0 cm^3/rev  Dv_nominal_specify=off  Dv_nominal_unit=cm^3/rev  Dv_nominal_value=1  dp_specify=off  dp_priority=None  dp=0 Pa  dp_nominal_specify=off  dp_nominal_unit=Pa  dp_nominal_value=1  we_specify=off  we_priority=None  we=0 rad/s  we_nominal_specify=off  we_nominal_unit=rad/s  we_nominal_value=1
      settings: InternalSimscapePortConfiguration="{\"Bottom\":[],\"Left\":[{\"id\":\"Vd\",\"label\":\"Vd\",\"type\":\"input\"},{\"id\":\"C\",\"label\":\"C\",\"type\":\"foundation.mechanical.rotational.rotational\"}],\"Right\":[{\"id\":\"A\",\"label\":\"A\",\"type\":\"foundation.hydraulic.hydraulic\"},{\"id\":\"B\",\"label\":\"B\",\"type\":\"foundation.hydraulic.hydraulic\"}],\"Top\":[]}"
  flexible shaft2 : flexshaft_lib/flexible shaft  b1=b1 N*m/(rad/s)  J1=J1 kg*m^2  b2=b2 N*m/(rad/s)  J2=J2 kg*m^2  b_theta=b_theta N*m/(rad/s)  k_theta=k_theta N*m/rad  w_1_specify=off  w_1_priority=None  w_1=0 rad/s  w_1_nominal_specify=off  w_1_nominal_unit=rad/s  w_1_nominal_value=1  w_2_specify=off  w_2_priority=None  w_2=0 rad/s  w_2_nominal_specify=off  w_2_nominal_unit=rad/s  w_2_nominal_value=1  t_1_specify=off  t_1_priority=None  t_1=0 N*m  t_1_nominal_specify=off  t_1_nominal_unit=N*m  t_1_nominal_value=1  t_2_specify=off  t_2_priority=None  t_2=0 N*m  t_2_nominal_specify=off  t_2_nominal_unit=N*m  t_2_nominal_value=1  t_theta_specify=off  t_theta_priority=None  t_theta=0 N*m  t_theta_nominal_specify=off  t_theta_nominal_unit=N*m  t_theta_nominal_value=1
      settings: InternalSimscapePortConfiguration="{\"Bottom\":[],\"Left\":[{\"id\":\"S1\",\"label\":\"S1\",\"type\":\"foundation.mechanical.rotational.rotational\"}],\"Right\":[{\"id\":\"S2\",\"label\":\"S2\",\"type\":\"foundation.mechanical.rotational.rotational\"},{\"id\":\"tau2\",\"label\":\"tau2\",\"type\":\"output\"},{\"id\":\"w2\",\"label\":\"w2\",\"type\":\"output\"}],\"Top\":[]}"
  pressure_charge_system_RD : Subsystem
      settings: PortSchema="{\"entries\":[{\"content\":{\"sides\":[{\"content\":{\"connectorIds\":[]},\"type\":\"ConnectorPlacement.EquallySpacedRectSide\",\"uuid\":\"e48dc60c-7abd-410a-894b-273047c8aadd\"},{\"content\":{\"connectorIds\":[],\"side\":\"RIGHT\"},\"type\":\"ConnectorPlacement.EquallySpacedRectSide\",\"uuid\":\"1866d745-b28e-4187-be81-03bff766c239\"},{\"content\":{\"connectorIds\":[\"LConn1\"],\"side\":\"TOP\"},\"type\":\"ConnectorPlacement.EquallySpacedRectSide\",\"uuid\":\"a7856f22-1a7f-4c46-a37a-59c4b01a6b79\"},{\"content\":{\"connectorIds\":[\"RConn1\",\"RConn2\"],\"side\":\"BOTTOM\"},\"type\":\"ConnectorPlacement.EquallySpacedRectSide\",\"uuid\":\"6254cc6e-0892-4919-86d5-0180151530d1\"}]},\"type\":\"ConnectorPlacement.EquallySpacedConnector\",\"uuid\":\"a983534e-afc0-4bb2-9b1c-06b03353b26b\"}],\"packageUris\":[\"http://schema.mathworks.com/mf0/Connector/19700101\"],\"version\":\"1.0\"}"
  vd_ctrl_motor_RD : Subsystem
  vd_ctrl_pump_RD : Subsystem
  s : PMIOPort  Side=Left
  q : PMIOPort  Port=2  Side=Right
  dp : PMIOPort  Port=3  Side=Right
  c : PMIOPort  Port=4  Side=Right
  pS1 : PMIOPort  Port=5  Side=Left
  pS2 : PMIOPort  Port=6  Side=Left
  pT1 : PMIOPort  Port=7  Side=Left
  pT2 : PMIOPort  Port=8  Side=Left
  RDA : PMIOPort  Port=9  Side=Right
  RDB : PMIOPort  Port=10  Side=Right
  wires:
  [DmA] -> vd_ctrl_motor_RD/1(vd_ref)
  [DpA] -> Gain1/1
  Gain1/1 -> vd_ctrl_pump_RD/1(vd_ref)
  connections:
  pT2/RConn1 -- Connection Label4/LConn1
  pS2/RConn1 -- Connection Label3/LConn1
  pT1/RConn1 -- Connection Label2/LConn1
  pS1/RConn1 -- Connection Label1/LConn1
  Variable displacement motor RD/RConn3 -- dp/RConn1
  Variable displacement motor RD/RConn1 -- c/RConn1
  Variable displacement motor RD/RConn2 -- q/RConn1
  s/RConn1 -- flexible shaft2/LConn1
  vd_ctrl_pump_RD/RConn1 -- Variable displacement pump RD/LConn1
  pressure_charge_system_RD/LConn1 -- RDA/RConn1 -- Variable displacement pump RD/RConn1 -- Variable displacement motor RD/LConn2
  vd_ctrl_motor_RD/LConn1 -- Connection Label8/LConn1
  vd_ctrl_motor_RD/LConn2 -- Connection Label9/LConn1
  vd_ctrl_motor_RD/RConn1 -- Variable displacement motor RD/LConn1
  Connection Label6/LConn1 -- vd_ctrl_pump_RD/LConn1
  Variable displacement pump RD/LConn2 -- pressure_charge_system_RD/RConn2 -- flexible shaft2/RConn1
  Connection Label7/LConn1 -- vd_ctrl_pump_RD/LConn2
  pressure_charge_system_RD/RConn1 -- Variable displacement motor RD/LConn3 -- RDB/RConn1 -- Variable displacement pump RD/RConn2

== system hdv_hydroelectropowertrain_model/PR776_powertrain/constant_pressure_source/Pressure controlled pump ==
  Hydraulic Flow Rate Sensor : fl_lib/Hydraulic/Hydraulic Sensors/Hydraulic Flow Rate Sensor
  Hydraulic Pressure Sensor : fl_lib/Hydraulic/Hydraulic Sensors/Hydraulic Pressure Sensor
  Hydraulic Reference : fl_lib/Hydraulic/Hydraulic Elements/Hydraulic Reference
  PS Step : fl_lib/Physical Signals/Sources/PS Step  step_time=20 s  initial_value=32 bar  final_value=32 bar
  PS-Simulink Converter : nesl_utility/PS-Simulink Converter  PhysicalDomain=network_engine_domain  SubClassName=ps_output  LeftPortType=input  RightPortType=output  PseudoPeriodic=off  Frequencies=[]  VectorFormat=1-D array  Unit=bar  AffineConversion=on
  PS-Simulink Converter1 : nesl_utility/PS-Simulink Converter  PhysicalDomain=network_engine_domain  SubClassName=ps_output  LeftPortType=input  RightPortType=output  PseudoPeriodic=off  Frequencies=[]  VectorFormat=1-D array  Unit=l/min  AffineConversion=on
  PS-Simulink Converter{2..5} (4 alike) : nesl_utility/PS-Simulink Converter  PhysicalDomain=network_engine_domain  SubClassName=ps_output  LeftPortType=input  RightPortType=output  PseudoPeriodic=off  Frequencies=[]  VectorFormat=1-D array  Unit=1  AffineConversion=off
  Pressure controlled pump : pressure_controlled_pump_lib/Pressure controlled pump  Vd_nom=62.3 cm^3/rev  pnom=32 bar  b=0.1 N*m/(rad/s)  inertia_pump=0.027 kg*m^2  vd_lim_max=0.98  vd_lim_min=0  p_set=258 bar  p_reg=8 bar  x_rv_max=12 mm  kpc=2  kic=40 1/s  te_specify=off  te_priority=None  te=0 N*m  te_nominal_specify=off  te_nominal_unit=N*m  te_nominal_value=1  qA_specify=off  qA_priority=None  qA=0 m^3/s  qA_nominal_specify=off  qA_nominal_unit=m^3/s  qA_nominal_value=1  qB_specify=off  qB_priority=None  qB=0 m^3/s  qB_nominal_specify=off  qB_nominal_unit=m^3/s  qB_nominal_value=1  qd_specify=off  qd_priority=None  qd=0 m^3/s  qd_nominal_specify=off  qd_nominal_unit=m^3/s  qd_nominal_value=1  dp_specify=off  dp_priority=None  dp=0 Pa  dp_nominal_specify=off  dp_nominal_unit=Pa  dp_nominal_value=1  vd_specify=off  vd_priority=None  vd=0  vd_nominal_specify=off  vd_nominal_unit=1  vd_nominal_value=1  vd_i_specify=off  vd_i_priority=None  vd_i=0  vd_i_nominal_specify=off  vd_i_nominal_unit=1  vd_i_nominal_value=1  we_specify=off  we_priority=None  we=0 rad/s  we_nominal_specify=off  we_nominal_unit=rad/s  we_nominal_value=1
      settings: InternalSimscapePortConfiguration="{\"Bottom\":[],\"Left\":[{\"id\":\"cW\",\"label\":\"cW\",\"type\":\"foundation.mechanical.rotational.rotational\"},{\"id\":\"dp_ref\",\"label\":\"Pressure set-point\",\"type\":\"input\"}],\"Right\":[{\"id\":\"cA\",\"label\":\"cA\",\"type\":\"foundation.hydraulic.hydraulic\"},{\"id\":\"cB\",\"label\":\"cB\",\"type\":\"foundation.hydraulic.hydraulic\"},{\"id\":\"qleak\",\"label\":\"qleak\",\"type\":\"output\"},{\"id\":\"taup\",\"label\":\"taup\",\"type\":\"output\"},{\"id\":\"vdi\",\"label\":\"vdi\",\"type\":\"output\"},{\"id\":\"pflow\",\"label\":\"pflow\",\"type\":\"output\"}],\"Top\":[]}"
  flow : Scope
  leak/ptorque : Scope  NumInputPorts=3
  pressure : Scope
  pump_flow : Scope
  pS : PMIOPort  Side=Right
  shaft : PMIOPort  Port=2  Side=Left
  pT : PMIOPort  Port=3  Side=Right
  wires:
  PS-Simulink Converter/1 -> pressure/1
  PS-Simulink Converter2/1 -> leak/ptorque/1  "leak"
  PS-Simulink Converter5/1 -> pump_flow/1
  PS-Simulink Converter3/1 -> leak/ptorque/2  "torque"
  PS-Simulink Converter4/1 -> leak/ptorque/3  "vd"
  PS-Simulink Converter1/1 -> flow/1
  connections:
  PS-Simulink Converter/LConn1 -- Hydraulic Pressure Sensor/RConn2
  Pressure controlled pump/RConn6 -- PS-Simulink Converter5/LConn1
  Pressure controlled pump/RConn5 -- PS-Simulink Converter4/LConn1
  Pressure controlled pump/RConn1 -- Hydraulic Flow Rate Sensor/LConn1
  Hydraulic Pressure Sensor/RConn1 -- pT/RConn1 -- Pressure controlled pump/RConn2 -- Hydraulic Reference/LConn1
  Hydraulic Flow Rate Sensor/RConn2 -- pS/RConn1 -- Hydraulic Pressure Sensor/LConn1
  Hydraulic Flow Rate Sensor/RConn1 -- PS-Simulink Converter1/LConn1
  Pressure controlled pump/RConn3 -- PS-Simulink Converter2/LConn1
  Pressure controlled pump/RConn4 -- PS-Simulink Converter3/LConn1
  shaft/RConn1 -- Pressure controlled pump/LConn1
  PS Step/RConn1 -- Pressure controlled pump/LConn2
